simulink model "hw"  (R2022b)
settings: Solver=VariableStepAuto  StartTime=0.0  StopTime=0.05  RelTol=1e-3
libraries: spsCurrentMeasurementLib x5, spsSeriesRLCBranchLib x5, spsVoltageMeasurementLib x4, spsMeanLib x2, spsDCVoltageSourceLib x1, spsDiodeLib x1, spsMosfetLib x1, spsVariableRatioTransformerLib x1, sps_lib x1
settings Model: Creator=tunaa  LastModifiedBy=Ekin Arda Çömez

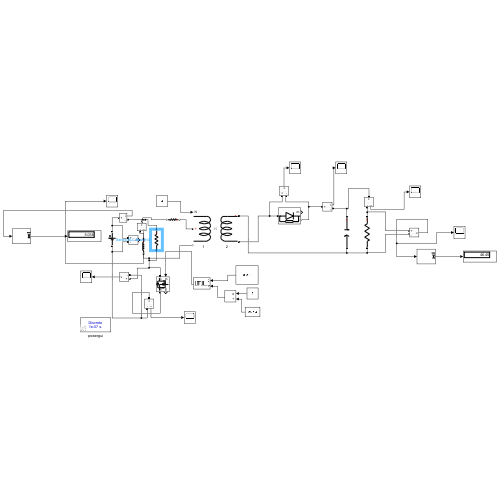
[thumbnail: Simulink's stored preview of the top-level diagram]
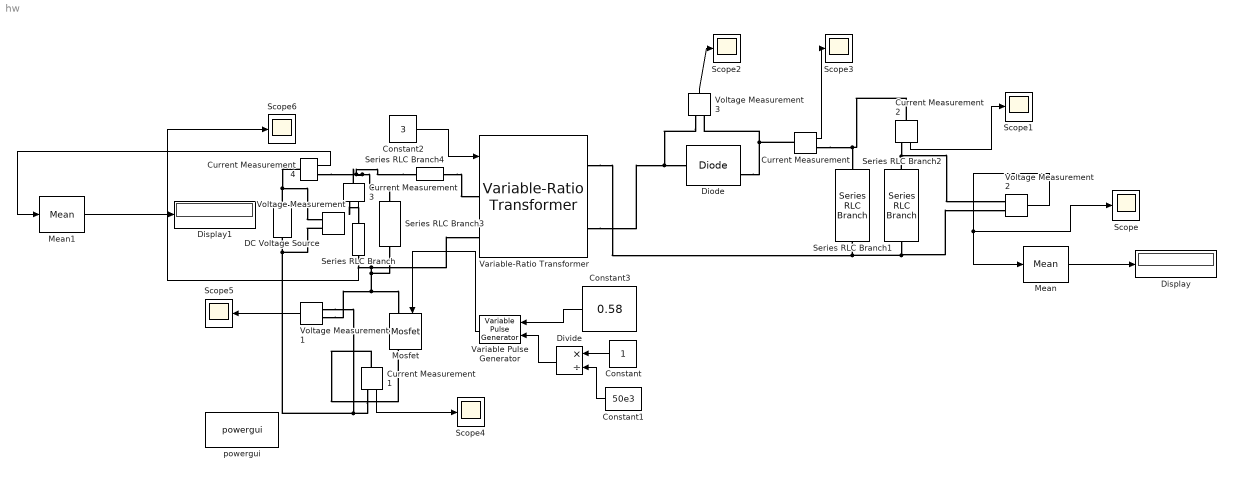
== system hw ==
  Constant : Constant
  Constant1 : Constant  Value=50e3
  Constant2 : Constant  Value=3
  Constant3 : Constant  Value=0.58
  Current Measurement{,1..4} (5 alike) : spsCurrentMeasurementLib/Current Measurement  PhasorSimulation=off  OutputType=Complex  PSBequivalent=0
  DC Voltage Source : spsDCVoltageSourceLib/DC Voltage Source  Amplitude=12  Measurements=None
  Diode : spsDiodeLib/Diode  Ron=0.001  Lon=0  Vf=0.8  IC=0  UseSnubber=0  Rs=500  Cs=250e-9  Measurements=on
  Display : Display
  Display1 : Display
  Divide : Product  Inputs=*/
  Mean : spsMeanLib/Mean  Freq=50000  Vinit=0  Ts=0
  Mean1 : spsMeanLib/Mean  Freq=50000  Vinit=0  Ts=0
  Mosfet : spsMosfetLib/Mosfet  Ron=0.044  Lon=0  Rd=0.01  Vfd=0  IC=0  Rs=1e5  Cs=inf  Measurements=on
  Scope{,1..6} (7 alike) : Scope
  Series RLC Branch : spsSeriesRLCBranchLib/Series RLC Branch  LConnTagsString=__new0  RConnTagsString=__new0  BranchType=L  Resistance=1  Inductance=59.68e-6  SetiL0=off  InitialCurrent=0  Capacitance=1e-6  Setx0=off  InitialVoltage=0  Measurements=None
  Series RLC Branch1 : spsSeriesRLCBranchLib/Series RLC Branch  LConnTagsString=__new0  RConnTagsString=__new0  BranchType=C  Resistance=1  Inductance=1e-3  SetiL0=off  InitialCurrent=0  Capacitance=10e-6  Setx0=off  InitialVoltage=0  Measurements=None
  Series RLC Branch2 : spsSeriesRLCBranchLib/Series RLC Branch  LConnTagsString=__new0  RConnTagsString=__new0  BranchType=R  Resistance=48  Inductance=1e-3  SetiL0=off  InitialCurrent=0  Capacitance=1e-6  Setx0=off  InitialVoltage=0  Measurements=None
  Series RLC Branch3 : spsSeriesRLCBranchLib/Series RLC Branch  LConnTagsString=__new0  RConnTagsString=__new0  BranchType=R  Resistance=21.57  Inductance=1e-3  SetiL0=off  InitialCurrent=0  Capacitance=1e-6  Setx0=off  InitialVoltage=0  Measurements=None
  Series RLC Branch4 : spsSeriesRLCBranchLib/Series RLC Branch  LConnTagsString=__new0  RConnTagsString=__new0  BranchType=R  Resistance=0.0389  Inductance=1e-3  SetiL0=off  InitialCurrent=0  Capacitance=1e-6  Setx0=off  InitialVoltage=0  Measurements=None
  Variable Pulse Generator : VariablePulseGenerator  SampleTime=0.1
  Variable-Ratio Transformer : spsVariableRatioTransformerLib/Variable-Ratio Transformer
      settings: LibrarySourceBlock=|
      | sps_lib/Passives/Variable-Ratio
      | Transformer
  Voltage Measurement{,1..3} (4 alike) : spsVoltageMeasurementLib/Voltage Measurement  PhasorSimulation=off  OutputType=Complex  PSBequivalent=0
  powergui : sps_lib/powergui  Priority=1  SimulationMode=Discrete  SampleTime=1e-7  frequency=60  Iterations=50  frequencyindice=0  Pbase=100e6  ErrMax=1e-4  UnitsV=kV  UnitsW=MW  buscounter=0  FunctionMessages=off  echomessages=off  EnableUseOfTLC=off  CurrentSourceSwitches=off  DisableSnubberDevices=off  DisableRonSwitches=off  DisableVfSwitches=off  DisplayEquations=off  AutomaticDiscreteSolvers=off  SolverType=Tustin/Backward Euler (TBE)  Interpol=off  ExternalGateDelay=off  methode=off  Ts=100  x0status=blocks  SPID=on  SwTol=0  HookPort=off  NonlinearTolerance=1e-4  nMaxIteration=100  ContinueOnMaxIteration=off  RestoreLinks=warning  ResistiveCurrentMeasurement=off  Frange=[0:2:500]  Ylog=off  Xlog=on  ShowGrid=off  save=off  variable=ZData  structure=0  ZoomFFT=off  StartTime=0.0  cycles=1  DisplayStyle=1  fundamental=60  FreqAxis=off  MaxFrequency=1000  frequencyindicesteady=1  RmsSteady=1  display=off
  wires:
  Variable Pulse Generator/1 -> Mosfet/1
  Constant/1 -> Divide/1
  Constant1/1 -> Divide/2
  Divide/1 -> Variable Pulse Generator/2
  Constant2/1 -> Variable-Ratio Transformer/1
  Voltage Measurement2/1 -> Mean/1, Scope/1
  Mean/1 -> Display/1
  Constant3/1 -> Variable Pulse Generator/1
  Current Measurement2/1 -> Scope1/1
  Voltage Measurement3/1 -> Scope2/1
  Current Measurement/1 -> Scope3/1
  Current Measurement1/1 -> Scope4/1
  Voltage Measurement1/1 -> Scope5/1
  Current Measurement3/1 -> Scope6/1
  Current Measurement4/1 -> Mean1/1
  Mean1/1 -> Display1/1
  connections:
  Series RLC Branch/RConn1 -- Voltage Measurement1/LConn1 -- Mosfet/LConn1 -- Series RLC Branch3/RConn1 -- Variable-Ratio Transformer/LConn2
  Variable-Ratio Transformer/RConn2 -- Voltage Measurement3/LConn1 -- Diode/LConn1
  Series RLC Branch2/LConn1 -- Current Measurement2/RConn1 -- Voltage Measurement2/LConn1
  Series RLC Branch2/RConn1 -- Voltage Measurement2/LConn2 -- Variable-Ratio Transformer/RConn1 -- Series RLC Branch1/RConn1
  Voltage Measurement/LConn2 -- Current Measurement1/RConn1 -- Voltage Measurement1/LConn2 -- DC Voltage Source/LConn1
  Current Measurement1/LConn1 -- Mosfet/RConn1
  Diode/RConn1 -- Current Measurement/LConn1 -- Voltage Measurement3/LConn2
  Current Measurement/RConn1 -- Current Measurement2/LConn1 -- Series RLC Branch1/LConn1
  Series RLC Branch4/LConn1 -- Variable-Ratio Transformer/LConn1
  DC Voltage Source/RConn1 -- Current Measurement4/LConn1 -- Voltage Measurement/LConn1
  Current Measurement3/RConn1 -- Series RLC Branch/LConn1
  Series RLC Branch4/RConn1 -- Current Measurement3/LConn1 -- Series RLC Branch3/LConn1 -- Current Measurement4/RConn1
